simulink model "FM"  (R2023b)
settings: Solver=VariableStepAuto  StartTime=0.0  StopTime=2  RelTol=1e-3
values from neighbouring files (symbols this model uses):
  ts_mux = 1/fs_mux    (= 3.33333333333e-06)    [simulink_parametros.m]
libraries: commanapbnd3 x2
settings Model: Creator=RomaW11  LastModifiedBy=RomaW11

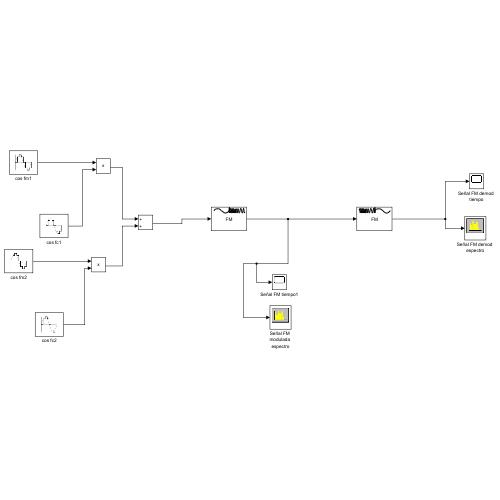
[thumbnail: Simulink's stored preview of the top-level diagram]
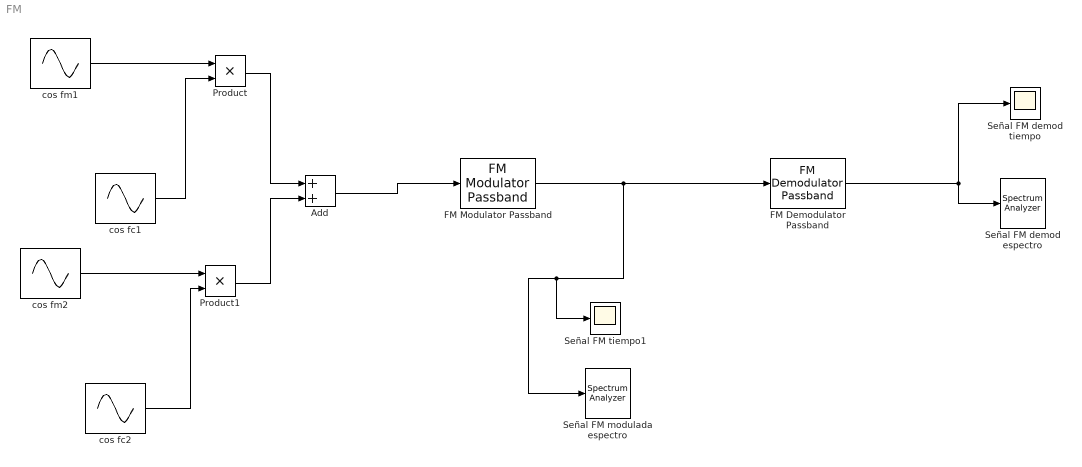
== system FM ==
  Add : Sum
  FM Demodulator Passband : commanapbnd3/FM Demodulator Passband  Fc=100  Ph=0  Kc=50  Ho=100
  FM Modulator Passband : commanapbnd3/FM Modulator Passband  Fc=5000  Ph=0  Kc=50
  Product : Product
  Product1 : Product
  Señal FM modulada espectro : SpectrumAnalyzer  WindowPosition=[1.000000,1.000000,1920.000000,1057.000000,]  ScopeFrameLocation=window  SampleRate=44.1e3  StartFrequency=20  StopFrequency=20e3  YLimits=[-254.73110184,54.94742733]  ShowLegend=on
      settings: OpenAtSimulationStart=off
  Señal FM demod espectro : SpectrumAnalyzer  WindowPosition=[1.000000,1.000000,1920.000000,1057.000000,]  ScopeFrameLocation=window  SampleRate=44.1e3  StartFrequency=20  StopFrequency=20e3  YLimits=[-69.60389106,27.43586964]  ShowLegend=on
      settings: OpenAtSimulationStart=off
  Señal FM demod tiempo : Scope
  Señal FM tiempo1 : Scope
  cos fc1 : Sin  Frequency=2*pi*100  Phase=pi/2  SampleTime=ts_mux
  cos fc2 : Sin  Frequency=2*pi*500  Phase=pi/2  SampleTime=ts_mux
  cos fm1 : Sin  Frequency=2*pi*10  Phase=pi/2  SampleTime=ts_mux
  cos fm2 : Sin  Frequency=2*pi*50  Phase=pi/2  SampleTime=ts_mux
  wires:
  FM Demodulator Passband/1 -> Señal FM demod tiempo/1, Señal FM demod espectro/1
  FM Modulator Passband/1 -> FM Demodulator Passband/1, Señal FM modulada espectro/1, Señal FM tiempo1/1
  cos fm1/1 -> Product/1
  cos fc1/1 -> Product/2
  cos fc2/1 -> Product1/2
  cos fm2/1 -> Product1/1
  Product/1 -> Add/1
  Add/1 -> FM Modulator Passband/1
  Product1/1 -> Add/2
